simulink model "test_yL_epsL"  (Simulink 7.9)
settings: Solver=ode23  StartTime=0.0  StopTime=tend  FixedStep=0.01  RelTol=1e-3
values from neighbouring files (symbols this model uses):
  delta = @(u) 0.0015*(u-t0)*(u>t0) - 0.0035*(u-t1)*(u>t1)    [test_yL_epsL_.m]
undefined symbols (not defined in the file or in its folder): pin
libraries: library x6, simulink x2, simulink_extras x1
settings Model: Creator=Georg  LastModifiedBy=georgnestlinger
settings OptimizationCC: InlineParams=on
settings DebuggingCC: SolverPrmCheckMsg=none  FcnCallInpInsideContextMsg=Use local settings
settings GRTTargetCC: CombineOutputUpdateFcns=off  GRTInterface=on

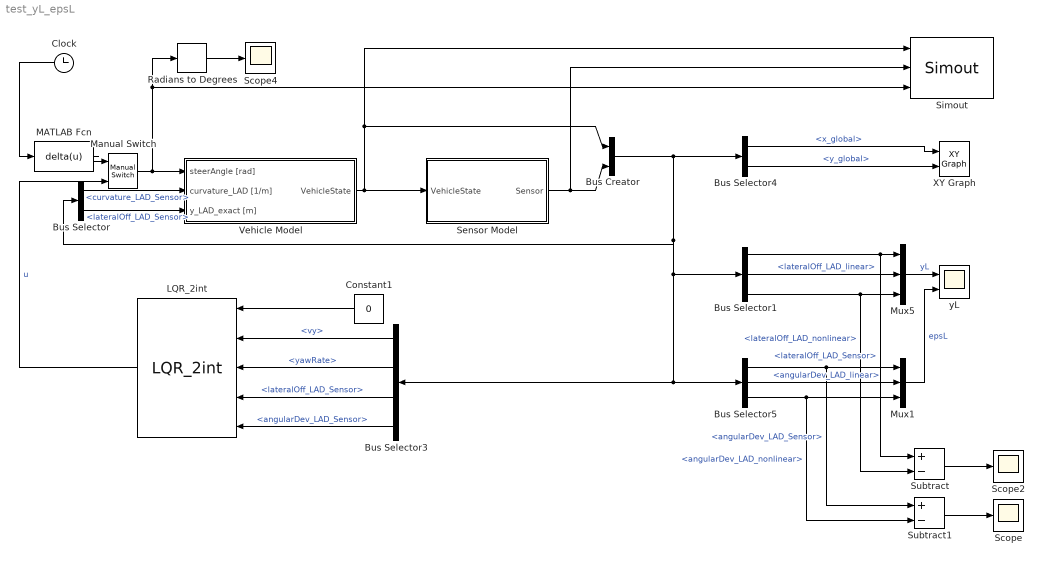
== system test_yL_epsL ==
  Bus Creator : BusCreator  Inputs=2
  Bus Selector : BusSelector  OutputSignals=LaneSensor.curvature_LAD_Sensor,LaneSensor.lateralOff_LAD_Sensor
  Bus Selector1 : BusSelector  OutputSignals=LaneSensor.lateralOff_LAD_Sensor,VehicleState.lateralOff_LAD_linear,VehicleState.lateralOff_LAD_nonlinear
  Bus Selector3 : BusSelector  OutputSignals=VehicleState.vy,VehicleState.yawRate,LaneSensor.lateralOff_LAD_Sensor,LaneSensor.angularDev_LAD_Sensor
  Bus Selector4 : BusSelector  OutputSignals=VehicleState.x_global,VehicleState.y_global
  Bus Selector5 : BusSelector  OutputSignals=LaneSensor.angularDev_LAD_Sensor,VehicleState.angularDev_LAD_linear,VehicleState.angularDev_LAD_nonlinear
  Clock : Clock
  Constant1 : Constant  Value=0
  LQR_2int : library/LKA-Controller/LQR_2int
  MATLAB Fcn : MATLABFcn  MATLABFcn=delta(u)
  Manual Switch : simulink/Signal Routing/Manual Switch  sw=1  action=0  varsize=off
  Mux1 : Mux  Inputs=3
  Mux5 : Mux  Inputs=3
  Radians to Degrees : simulink_extras/Transformations/Radians to Degrees
  Scope : Scope
  Scope2 : Scope
      settings: SaveName=ScopeData4
  Scope4 : Scope
      settings: YMin=-0.4  YMax=1.1
  Sensor Model : Subsystem
  Simout : library/Misc/Simout
  Subtract : Sum  Inputs=+-
  Subtract1 : Sum  Inputs=+-
  Vehicle Model : Subsystem
  XY Graph : simulink/Sinks/XY Graph  xmin=-50  xmax=700  ymin=-10  ymax=600  st=-1
  yL : Scope  NumInputPorts=2
      settings: ShowLegends=on  TimeRange=28  YMin=-0.325~-5  YMax=0~5  SaveName=ScopeData3
  wires:
  Bus Selector4/1 -> XY Graph/1  "<x_global>"
  Bus Selector4/2 -> XY Graph/2  "<y_global>"
  Sensor Model/1(Sensor) -> Simout/2, Bus Creator/2
  Bus Creator/1 -> Bus Selector4/1, Bus Selector5/1, Bus Selector3/1, Bus Selector1/1, Bus Selector/1
  Vehicle Model/1(VehicleState) -> Sensor Model/1(VehicleState), Bus Creator/1, Simout/1
  Constant1/1 -> LQR_2int/1
  Bus Selector3/1 -> LQR_2int/2  "<vy>"
  Bus Selector3/2 -> LQR_2int/3  "<yawRate>"
  Bus Selector3/3 -> LQR_2int/4  "<lateralOff_LAD_Sensor>"
  Bus Selector3/4 -> LQR_2int/5  "<angularDev_LAD_Sensor>"
  LQR_2int/1 -> Manual Switch/2  "u"
  MATLAB Fcn/1 -> Manual Switch/1
  Manual Switch/1 -> Radians to Degrees/1, Simout/3, Vehicle Model/1(steerAngle [rad])
  Bus Selector1/1 -> Mux5/1, Subtract/1  "<lateralOff_LAD_Sensor>"
  Bus Selector1/2 -> Mux5/2  "<lateralOff_LAD_linear>"
  Clock/1 -> MATLAB Fcn/1
  Radians to Degrees/1 -> Scope4/1
  Bus Selector5/1 -> Mux1/1, Subtract1/1  "<angularDev_LAD_Sensor>"
  Bus Selector5/2 -> Mux1/2  "<angularDev_LAD_linear>"
  Bus Selector5/3 -> Mux1/3, Subtract1/2  "<angularDev_LAD_nonlinear>"
  Bus Selector1/3 -> Mux5/3, Subtract/2  "<lateralOff_LAD_nonlinear>"
  Subtract1/1 -> Scope/1
  Mux1/1 -> yL/2  "epsL"
  Mux5/1 -> yL/1  "yL"
  Subtract/1 -> Scope2/1
  Bus Selector/1 -> Vehicle Model/2(curvature_LAD [1/m])  "<curvature_LAD_Sensor>"
  Bus Selector/2 -> Vehicle Model/3(y_LAD_exact [m])  "<lateralOff_LAD_Sensor>"

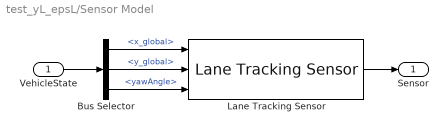
== system test_yL_epsL/Sensor Model ==
  VehicleState : Inport
  Bus Selector : BusSelector  OutputSignals=x_global,y_global,yawAngle
  Lane Tracking Sensor : library/Lane Tracking/Lane Tracking Sensor
  Sensor : Outport
  wires:
  Lane Tracking Sensor/1 -> Sensor/1
  VehicleState/1 -> Bus Selector/1
  Bus Selector/1 -> Lane Tracking Sensor/1  "<x_global>"
  Bus Selector/2 -> Lane Tracking Sensor/2  "<y_global>"
  Bus Selector/3 -> Lane Tracking Sensor/3  "<yawAngle>"

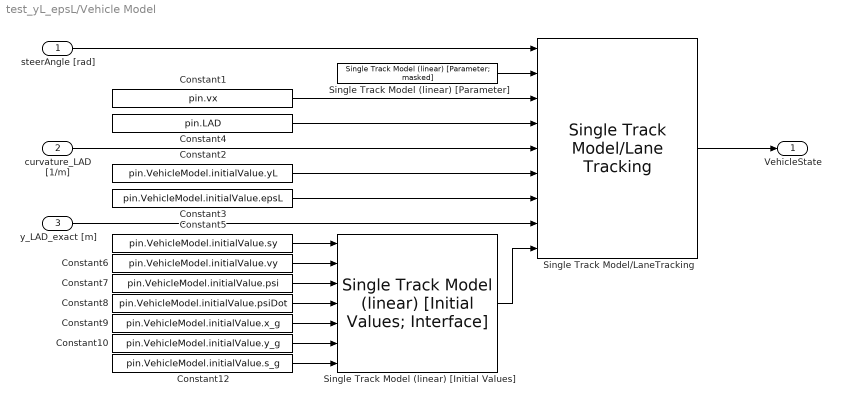
== system test_yL_epsL/Vehicle Model ==
  steerAngle [rad] : Inport
  curvature_LAD [1/m] : Inport  Port=2
  y_LAD_exact [m] : Inport  Port=3
  Constant1 : Constant  Value=pin.vx
  Constant10 : Constant  Value=pin.VehicleModel.initialValue.y_g
  Constant12 : Constant  Value=pin.VehicleModel.initialValue.s_g
  Constant2 : Constant  Value=pin.VehicleModel.initialValue.yL
  Constant3 : Constant  Value=pin.VehicleModel.initialValue.epsL
  Constant4 : Constant  Value=pin.LAD
  Constant5 : Constant  Value=pin.VehicleModel.initialValue.sy
  Constant6 : Constant  Value=pin.VehicleModel.initialValue.vy
  Constant7 : Constant  Value=pin.VehicleModel.initialValue.psi
  Constant8 : Constant  Value=pin.VehicleModel.initialValue.psiDot
  Constant9 : Constant  Value=pin.VehicleModel.initialValue.x_g
  Single Track Model (linear) [Initial Values] : library/Vehicle Models ext./Single Track Model (linear) [Initial Values; Interface]
  Single Track Model (linear) [Parameter] : library/Vehicle Models ext./Single Track Model (linear) [Parameter; masked]  cs_front=pin.VehicleModel.parameter.csv  cs_rear=pin.VehicleModel.parameter.csh  l_front=pin.VehicleModel.parameter.lv  l_rear=pin.VehicleModel.parameter.lh  m=pin.VehicleModel.parameter.m  Izz=pin.VehicleModel.parameter.Iz
  Single Track Model/LaneTracking : library/Vehicle Models ext./Single Track Model//Lane Tracking
  VehicleState : Outport
  wires:
  Single Track Model/LaneTracking/1 -> VehicleState/1
  Constant2/1 -> Single Track Model/LaneTracking/6
  Constant3/1 -> Single Track Model/LaneTracking/7
  Constant1/1 -> Single Track Model/LaneTracking/3
  Constant4/1 -> Single Track Model/LaneTracking/4
  steerAngle [rad]/1 -> Single Track Model/LaneTracking/1
  curvature_LAD [1/m]/1 -> Single Track Model/LaneTracking/5
  y_LAD_exact [m]/1 -> Single Track Model/LaneTracking/8
  Single Track Model (linear) [Parameter]/1 -> Single Track Model/LaneTracking/2
  Single Track Model (linear) [Initial Values]/1 -> Single Track Model/LaneTracking/9
  Constant5/1 -> Single Track Model (linear) [Initial Values]/1
  Constant6/1 -> Single Track Model (linear) [Initial Values]/2
  Constant7/1 -> Single Track Model (linear) [Initial Values]/3
  Constant8/1 -> Single Track Model (linear) [Initial Values]/4
  Constant9/1 -> Single Track Model (linear) [Initial Values]/5
  Constant10/1 -> Single Track Model (linear) [Initial Values]/6
  Constant12/1 -> Single Track Model (linear) [Initial Values]/7
